simulink model "CAN_Communication"  (Simulink 8.3)
settings: Solver=ode1  StartTime=0.0  StopTime=Inf  FixedStep=0.001  RelTol=1e-3
PostLoadFcn:
  | , if any(exist('dsrtsu_mdlpostloadfcn', 'file') == [2, 3, 6]), try dsrtsu_mdlpostloadfcn('Execute', bdroot); catch fprintf('Error in PostLoadFcn (dsrtsu_mdlpostloadfcn) for model "%s":\n %s\n', bdroot, lasterr); end, end,
undefined symbols (not defined in the file or in its folder): rticanmm_blockfcn, rticanmm_initfcn
libraries: rtimmsu_dsrtlib x2
settings Model: DSRTSU_INTERNAL_RTI_VER=440  DSRTSU_INTERNAL_RTI_TYPE=rti1401  RTICANMMDATA=struct('GeneralSetupData',struct('modelroot','C:\Users\Sebastian\Desktop\DBC_Files','generalsettings',struct('filesettings',struct('destfolder',struct('Name','RTICANMM_FILES','Check',1),'buildfolder',struct('Name','.','Check',1),'AbsDestfolder',struct('Name','C:\Users\Sebastian\Desktop\DBC_Files\RTICANMM_FILES'),'AbsBuildfolder',struct('Name','C:\Users\Sebastian\Desktop\DBC_Files'))),'options',struct('addpaths',1,'rmpaths',1,'addtrcexclusion',logical(1),'cannavigator',struct('checkmonitoring',0),'show_usrtrc',0,'use_usrtrc',0,'addpath2usrmk',1),'advanced',struct('options',[1 1 1 1 1 1 1 1 1 1 1 1 1 1 1 1 1 1 1 1 1 1 1 1 1 1 1 1 1 1 1 1 1 1 1 1 1 1 1 1 1 1 1 1 1 1 1 1 1 1 1 1 1 1 1 1 1 1 1 1 1 1 1 1 1 1 1 1 1 1 1 1 1 1 1 1 1 1 1 1 1 1 1 1 1 1 1 1 1 1 1 1 1 1 1 1 1 1 1 1]),'MPSetup',{{}},'modelname','CAN_Communication','blockdata',struct('generalsettings',struct('filesettings',struct('destfolder',struct('Name','.','Check',1),'AbsDestfolder',struct('Name','T:\TOOL_SOURCES\CANnedy\m'),'buildfolder',struct('Name','.','Check',1),'AbsBuildfolder',struct('Name','C:\MATLAB6p5\work'))),'options',struct('addpaths',1,'rmpaths',1,'addpath2usrmk',1),'modelname','rticanmmlib','modelroot','T:\TOOL_SOURCES\CANnedy\m'),'MMType','RTICANMM','block',['CAN_Communication/RTICANMM' char(10) 'GeneralSetup'],'RTI',struct('Type','RTI1401','Ver','7.2','Date','02-May-2014'),'version','3.0.735671.4434490741','userdata',struct('HostServiceChannelID',{{'Controller1'}})))  DSRTSU_INTERNAL_RTIFPGA=30  Creator=Sebastian  LastModifiedBy=Sebastian  BufferReuse=off
settings DataIOCC: SignalLoggingSaveFormat=Dataset
settings OptimizationCC: BlockReduction=off  OptimizeBlockIOStorage=off  BufferReuse=off  GlobalBufferReuse=off  ExpressionFolding=off  LocalBlockOutputs=off
settings DebuggingCC: StateNameClashWarn=none
settings HardwareCC: ProdIntDivRoundTo=Zero  ProdEndianess=BigEndian  ProdHWDeviceType=Generic->Custom  TargetIntDivRoundTo=Zero  TargetEndianess=BigEndian  TargetHWDeviceType=Generic->Custom
settings RTWCC: SystemTargetFile=rti1401.tlc  MakeCommand=make_rti  TemplateMakefile=rti1401.tmf  Description=dSPACE DS1401 Hardware Platform  ProcessScript=rti1401_make_rtw_hook
settings STFCustomTargetCC: ParMdlRefBuildCompliant=on  GeneratePreprocessorConditionals=Disable all  SystemTargetFile=rti1401.tlc
settings GRTTargetCC: CompOptLevelCompliant=off  ConcurrentExecutionCompliant=off  MatFileLogging=off  CPPClassGenCompliant=off  ExtModeMexFile=noextcomm
settings CustomProperty: DataType=RTWOptions_EnumType_C__Program Files_dSPACE RCPHIL 2014-A_MATLAB_RTI_RTI1401_TLC_rti1401_1InitialSimState  Value=RUN
settings EnumStrPairs: String=RUN

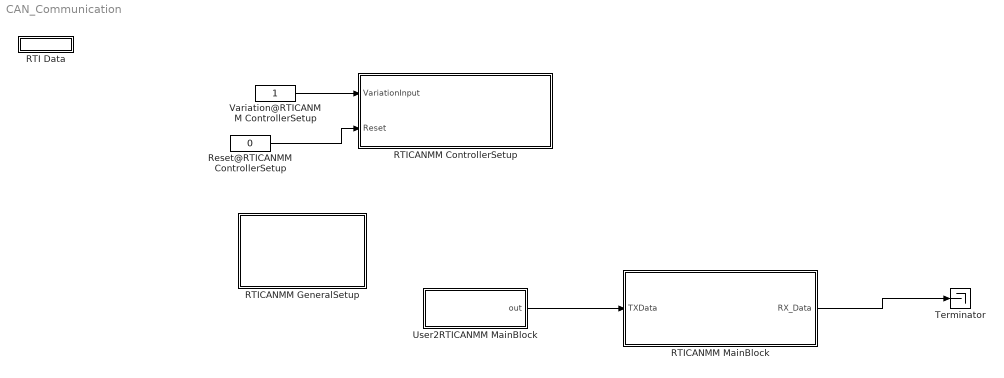
== system CAN_Communication ==
  RTI Data : Subsystem  Tag=struct('RTIDataServer',struct('RTIDataServerVs','2','RTIModelDescription','struct(''main'',''CAN_Communication'',''sub'','''',''isMp'',0)'))  LoadFcn="if exist('rtidc'), try,  rtidc('DataHostBlockClbLoad', gcbh); catch, disp(['Warning: ''LoadFcn'' for RTI Data block failed: ' lasterr]); end, end,"  mask(RTI_DATA_HOST){}
      mask help:
      | RTI Data Block.
      | This block is used by RTI to store internal model-dependent data.
      | Please keep this block on the root level of the model. Deleting this block will result in data loss.
      |
      | NEVER DELETE OR COPY THIS BLOCK!
      settings: CopyFcn="if exist('rtidc'), try,  rtidc('DataHostBlockClbCopy', gcbh); catch, disp(['Warning: ''CopyFcn'' for RTI Data block failed: ' lasterr]); end, end,"  DeleteFcn="if exist('rtidc'), try,  rtidc('DataHostBlockClbDelete', gcbh); catch, disp(['Warning: ''DeleteFcn'' for RTI Data block failed: ' lasterr]); end, end,"  ModelCloseFcn="if exist('rtidc'), try,  rtidc('DataHostBlockClbModelClose', gcbh); catch, disp(['Warning: ''ModelCloseFcn'' for RTI Data block failed: ' lasterr]); end, end,"  PreSaveFcn="if exist('rtidc'), try,  rtidc('DataHostBlockClbPreSave', gcbh); catch, disp(['Warning: ''PreSaveFcn'' for RTI Data block failed: ' lasterr]); end, end,"  PostSaveFcn="if exist('rtidc'), try,  rtidc('DataHostBlockClbPostSave', gcbh); catch, disp(['Warning: ''PostSaveFcn'' for RTI Data block failed: ' lasterr]); end, end,"  NameChangeFcn="if exist('rtidc'), try,  rtidc('DataHostBlockClbNameChange', gcbh); catch, disp(['Warning: ''NameChangeFcn'' for RTI Data block failed: ' lasterr]); end, end,"
      mask Help:
      | RTI Data Block.
      | This block is used by RTI to store internal model-dependent data.
      | Please keep this block on the root level of the model. Deleting this block will result in data loss.
      | 
      | NEVER DELETE OR COPY THIS BLOCK!
      mask Display:
      | text(0.5, 0.5, 'RTI Data', 'HorizontalAlignment', 'center');
      | plot([1 0]);
  RTICANMM ControllerSetup : Subsystem  InitFcn=rticanmm_blockfcn('InitFcn', 'CANnedySetup', gcb)  ClipboardFcn=rticanmm_blockfcn('ClipboardFcn', 'CANnedySetup', gcb)  mask(RTICANMM){DSProperties=struct('RTI',struct('Version',uint32(1),'BlockType',struct('isSLSource',uint8(1),'isSLSink',uint8(1),'isHWSource',uint8(0),'isHWSink',uint8(0),'isSetup',uint8(0),'isInline',uint8(1),'isNonInline',uint8(0),'isInterrupt',uint8(0),'isChannelwise',uint8(0)),'IOBoardType','RTICANMM','UnitType','RTICANMM','Identifier','BUSSETUP','DialogType','SL','BlockSet','RTICANMM','SlaveProcessor','CAN')), CANMMProperties=struct('cannedy',struct('data',struct('options',struct('controllername','Controller1','controllernameautomatic',[],'loglevel','0','checkrealtime',0,'checkchangebaudrate',0,'sampletime','1.000','CANControllerStatus',0,'NumberofStuffErr',0,'NumberofFormErr',0,'NumberofAckErr',0,'NumberofBit0Err',0,'NumberofsuccrecRX',0,'Numberofsuccsent',0,'NumberofBit1Err',0,'NumberofCRCErr',0,'NumberoflostRX',0,'Busoff',0,'Busload',0,'OperationPending',0,'TxRetryCount',3,'addtrcexclusion',logical(1),'cannavigator',struct('checkmonitoring',0,'checkinternmonitoring',0),'show_usrtrc',0,'use_usrtrc',0),'modelroot','C:\Users\Sebastian\Desktop\DBC_Files','generalsettings',struct('setupdata',struct('board',['CAN Type 1'],'boardno',1,'channelno',1,'Type','STD','transceiver','ISO11898-2','busconfig','0x0','feedthrough','false','resistance',struct('r120',1,'roff',0,'r16',1,'r10',0),'baudrate','500','Frequency',[24 36],'samplemode',1,'commChannelTJA1041',6,'config',struct('standard',1,'advanced',0,'register',struct('btr0','0xC0','btr1','0x6F','sp','70','sjw','3','tseg1','15','tseg2','6','brp','0','smpl','0','btr0_36','0x41','btr1_36','0x1E','sp_36','88','sjw_36','1','tseg1_36','14','tseg2_36','1','brp_36','1','smpl_36','0','btr0_64','0x43','btr1_64','0x1C','sp_64','87','sjw_64','1','tseg1_64','12','tseg2_64','1','brp_64','3','smpl_64','0')),'channelcfg',struct('INTENDISABLE','CAN_INT_DISABLE','intenable',0),'SETUPID','RTICANMM_Controller1_ID','CONTROLLER_ID','CANMM_CTL_SETUP_Controller1','mainblock_includefile','RTICANMM_SETUP_Controller1','termination','TERMINATION_ON'),'filesettings',struct('destfolder',struct('Name','RTICANMM_FILES','Check',1),'buildfolder',struct('Name','.','Check',1))),'advanced',struct('options',[1 1 1 1 1 1 1 1 1 1 1 1 1 1 1 1 1 1 1 1 1 1 1 1 1 1 1 1 1 1 1 1 1 1 1 1 1 1 1 1 1 1 1 1 1 1 1 1 1 1 1 1 1 1 1 1 1 1 1 1 1 1 1 1 1 1 1 1 1 1 1 1 1 1 1 1 1 1 1 1 1 1 1 1 1 1 1 1 1 1 1 1 1 1 1 1 1 1 1 1]),'partialnetdata',struct('switchedon',0,'format','STD','idmask',['XXXXX XXXXXXXX XXXXXXXX XXXXXXXX'],'idcode','0','idfilter','0','datamaskused',0,'datalength','0','datamask','0x0000000000000000','partialnetworkenable',0)),'blk',['CAN_Communication/RTICANMM' char(10) 'ControllerSetup'],'allgeneratedfiles',{{'C:\Users\Sebastian\Desktop\DBC_Files\RTICANMM_FILES\RTICANMM_SETUP_Controller1.c','C:\Users\Sebastian\Desktop\DBC_Files\RTICANMM_FILES\RTICANMM_SETUP_Controller1.h','c:\users\sebastian\desktop\dbc_files\rticanmm_files\rticanmm_setup_controller1.mexw64'}},'ismp',logical(0),'BlockDataVersion','0.6.0','recreate',0),'CANnedynew',0,'CANnedySettings','Controller1','GeneratedFiles',{{'C:\Users\Sebastian\Desktop\DBC_Files\RTICANMM_FILES\RTICANMM_SETUP_Controller1.c','C:\Users\Sebastian\Desktop\DBC_Files\RTICANMM_FILES\RTICANMM_SETUP_Controller1.h','c:\users\sebastian\desktop\dbc_files\rticanmm_files\rticanmm_setup_controller1.mexw64'}},'SFCN','RTICANMM_SETUP_Controller1.c','HostService',struct('Tags',struct('DATA','RTICANMM_MonitorData','Enable','CANMMMonitor_Controller1','TimeStamp','MonitoringTimeStamp_Controller1'),'DATA',struct('Length',4),'Info',struct('Desc',{'ID','Service','Data1','Data2'}),'Names',struct('Enable','Monitoring_Enable','TimeStamp','Monitoring_TimeStamp'),'ChannelID',1)), CANMMType=CANnedySetup, CANMMFolder=C:\Users\Sebastian\Desktop\DBC_Files, CANMMDestFolder=RTICANMM_FILES, CANMMSettings=Controller1, CANMMSFcn=RTICANMM_SETUP_Controller1, CANMMBoard=DS1401, CANMMBoardNum=1, CANMMChannel=1}
      settings: AttributesFormatString=%<CANMMSettings>: %<CANMMBoard>_B%<CANMMBoardNum>_C%<CANMMChannel>  CopyFcn=rticanmm_blockfcn('CopyFcn', 'CANnedySetup', gcb)  DeleteFcn=rticanmm_blockfcn('DeleteFcn', 'CANnedySetup', gcb)  ModelCloseFcn=rticanmm_blockfcn('ModelCloseFcn', 'CANnedySetup', gcb)  NameChangeFcn=rticanmm_blockfcn('NameChangeFcn', 'CANnedySetup', gcb)  OpenFcn=try, rticanmm_setup_gui('create',gcb); ; catch,errordlg({lasterr, '','Please check your RTI installation.'},['Error: ' upper(bdroot)], 'replace'); end  MoveFcn=rticanmm_blockfcn('MoveFcn', 'CANnedySetup', gcb)
      mask Help: eval('rticanmm_quickstart(''create'', gcb);', 'disp(lasterr);')
      mask Display:
      | disp('RTI CAN\nMultiMessage\nControllerSetup')
      | 
      | port_label('input', 1 , 'Variation')
      | port_label('input', 2 , 'Reset')
  RTICANMM GeneralSetup : Subsystem  InitFcn=rticanmm_initfcn(gcb, 'CANnedySettings')  ClipboardFcn=rticanmm_blockfcn('ClipboardFcn', 'CANnedySettings', gcb)  mask(RTICANMM){DSProperties=struct('RTI',struct('Version',uint32(1),'BlockType',struct('isSLSource',uint8(1),'isSLSink',uint8(1),'isHWSource',uint8(0),'isHWSink',uint8(0),'isSetup',uint8(0),'isInline',uint8(1),'isNonInline',uint8(0),'isInterrupt',uint8(0),'isChannelwise',uint8(0)),'IOBoardType','RTICANMM','UnitType','RTICANMM','Identifier','GENERALSETUP','DialogType','SL','BlockSet','RTICANMM','SlaveProcessor','CAN')), CANMMDestFolder=RTICANMM_FILES, CANMMBuildDir=., CANMMAddPaths=on, CANMMAddpathUserMake=on, CANMMRemovePathOnclose=on, CANMMType=CANnedySettings, CANMMProperties=struct('modelroot','C:\Users\Sebastian\Desktop\DBC_Files','generalsettings',struct('filesettings',struct('destfolder',struct('Name','RTICANMM_FILES','Check',1),'buildfolder',struct('Name','.','Check',1),'AbsDestfolder',struct('Name','C:\Users\Sebastian\Desktop\DBC_Files\RTICANMM_FILES'),'AbsBuildfolder',struct('Name','C:\Users\Sebastian\Desktop\DBC_Files'))),'options',struct('addpaths',1,'rmpaths',1,'addtrcexclusion',logical(1),'cannavigator',struct('checkmonitoring',0),'show_usrtrc',0,'use_usrtrc',0,'addpath2usrmk',1),'advanced',struct('options',[1 1 1 1 1 1 1 1 1 1 1 1 1 1 1 1 1 1 1 1 1 1 1 1 1 1 1 1 1 1 1 1 1 1 1 1 1 1 1 1 1 1 1 1 1 1 1 1 1 1 1 1 1 1 1 1 1 1 1 1 1 1 1 1 1 1 1 1 1 1 1 1 1 1 1 1 1 1 1 1 1 1 1 1 1 1 1 1 1 1 1 1 1 1 1 1 1 1 1 1]),'MPSetup',{{}},'modelname','CAN_Communication','blockdata',struct('generalsettings',struct('filesettings',struct('destfolder',struct('Name','.','Check',1),'AbsDestfolder',struct('Name','T:\TOOL_SOURCES\CANnedy\m'),'buildfolder',struct('Name','.','Check',1),'AbsBuildfolder',struct('Name','C:\MATLAB6p5\work'))),'options',struct('addpaths',1,'rmpaths',1,'addpath2usrmk',1),'modelname','rticanmmlib','modelroot','T:\TOOL_SOURCES\CANnedy\m'),'MMType','RTICANMM','block',['CAN_Communication/RTICANMM' char(10) 'GeneralSetup'],'RTI',struct('Type','RTI1401','Ver','7.2','Date','02-May-2014'),'version','3.0.735671.4434490741','userdata',struct('HostServiceChannelID',{{'Controller1'}}))}
      mask prompts: CANMMDestFolder "Destination Folder for generated Files:"; CANMMBuildDir "Build Directory (*_usr.mk, *_usr.trc)"; CANMMAddPaths "Add Paths automatically"; CANMMAddpathUserMake "Add Paths to UserMake-File"; CANMMRemovePathOnclose "Remove added Path on ModelClose"
      mask init:
      | rticanmm_initfcn(gcb,'CANnedyGeneralSettings')
      settings: CopyFcn=rticanmm_blockfcn('CopyFcn', 'CANnedySettings', gcb)  DeleteFcn=rticanmm_blockfcn('DeleteFcn', 'CANnedySettings', gcb)  ModelCloseFcn=rticanmm_blockfcn('CloseFcn', 'CANnedyGeneralSettings', gcb)  NameChangeFcn=rticanmm_blockfcn('NameChangeFcn', 'CANnedySettings', gcb)  OpenFcn=try, rticanmm_gs_gui('create',gcb), ; catch,errordlg({lasterr, '','Please check your RTI installation.'},['Error: ' upper(bdroot)], 'replace'); end  MoveFcn=rticanmm_blockfcn('MoveFcn', 'CANnedySettings', gcb)
      mask Help: eval('rticanmm_quickstart(''create'', gcb);', 'disp(lasterr);')
      mask Display: disp(sprintf(['RTI CAN\nMultiMessage\nGeneralSetup']))
  RTICANMM MainBlock : Subsystem  InitFcn=rticanmm_blockfcn('InitFcn', 'CANnedy', gcb)  ClipboardFcn=rticanmm_blockfcn('ClipboardFcn', 'CANnedy', gcb)  mask(RTICANMM){DSProperties=struct('RTI',struct('Version',uint32(1),'BlockType',struct('isSLSource',uint8(1),'isSLSink',uint8(1),'isHWSource',uint8(0),'isHWSink',uint8(0),'isSetup',uint8(0),'isInline',uint8(1),'isNonInline',uint8(0),'isInterrupt',uint8(0),'isChannelwise',uint8(0)),'IOBoardType','RTICANMM','UnitType','RTICANMM','Identifier','Mainblock','DialogType','SL','BlockSet','RTICANMM','SlaveProcessor','CAN')), CANMMProperties=struct('RTICANMMVersion','3.0','RTICANMMVersionIntern','3.0.735671.4434490741','RTICANMMDate','02-May-2014','Settings','RTICANMM_MAIN_CAN','UserTracePath','','ModelPath','C:\Users\Sebastian\Desktop\DBC_Files','filesettings',struct('FileName','AngleSpeed.dbc','IsRelative',1,'ClusterId',1,'ClusterList',{{'default'}},'destfolder',struct('Name','RTICANMM_FILES','Check',1),'buildfolder',struct('Name','.','Check',1),'onlyfreerawcapture',0,'overlapping2variant',0),'onlyfreerawcapture',0,'Board',['CAN Type 1'],'BoardNum','1','ChannelNum','1','Variation','1','SetupId','Controller1','MARK',['719753203727948A60AC430329C9D5';'48A0AF194FAB6FB27E8338C8940826';'1300DB01B7EF55C98D2EBFEB02253B';'5389981ECFCAA947711D2E68ACED04';'4C61CF917CD092FC8858619250CB50'],'date','13-Jan-2015','clock',['13.01.2015 19:24:34'],'recreate',0,'RTIVER','RTI1401','j1939',0,'TRC',struct('include',1),'rtsupport',struct('XMLFile','C:\Users\Sebastian\Desktop\DBC_Files\RTICANMM_FILES\RTICANMM_MAIN_CAN.xml','DBCXML',struct('Path','C:\Users\Sebastian\Desktop\DBC_Files\RTICANMM_FILES\RTICANMM_MAIN_CAN_dbc.xml','support',1,'Name','AngleSpeed.dbc','Date',['11-Dez-2014 10:18:45'],'Type','extended','DBCSupport','ON'))), CANMMType=CANnedy, CANMMUserTraceMerged=off, CANMMUserTracePath=, CANMMChannelNum=1, CANMMBoardNum=1, CANMMDestFolder=RTICANMM_FILES, CANMMFolder=., CANMMSetupId=Controller1, CANMMsave2mat=['719753203727948A60AC430329C9D5';'48A0AF194FAB6FB27E8338C8940826';'1300DB01B7EF55C98D2EBFEB02253B';'5389981ECFCAA947711D2E68ACED04';'4C61CF917CD092FC8858619250CB50'], CANMMName=CAN, CANMMSettings=RTICANMM_MAIN_CAN, CANMMIntermediateTag=RTICANMM_MAIN_CAN_intermediate, CANMMsfcnname=RTICANMM_MAIN_CAN}
      mask init:
      | rticanmm_initfcn(gcb, CANMMType, CANMMsfcnname)
      settings: AttributesFormatString=Controller1[CAN]: DS1401_B1_C1_V1  CopyFcn=rticanmm_blockfcn('CopyFcn', 'CANnedy', gcb)  DeleteFcn=rticanmm_blockfcn('DeleteFcn', 'CANnedy', gcb)  ModelCloseFcn=rticanmm_blockfcn('ModelCloseFcn', 'CANnedy', gcb)  NameChangeFcn=rticanmm_blockfcn('NameChangeFcn', 'CANnedy', gcb)  OpenFcn=try, rticanmm_main_gui('create',gcb); ; catch,errordlg({lasterr, '','Please check your RTI installation.'},['Error: ' upper(bdroot)], 'replace'); end  MoveFcn=rticanmm_blockfcn('MoveFcn', 'CANnedy', gcb)
      mask Help: eval('rticanmm_quickstart(''create'', gcb);', 'disp(lasterr);')
      mask Display:
      | disp(sprintf('RTI CAN\nMultiMessage\nMainSetup'))
      | port_label('input', 1, 'TX Data')
      | port_label('output', 1, 'RX Data')
  Reset@RTICANMM ControllerSetup : Constant  Value=0  OutDataTypeStr=boolean
  Terminator : Terminator
  User2RTICANMM MainBlock : Subsystem
      mask Display: disp('Mapping\nto RTICANMM')
  Variation@RTICANMM ControllerSetup : Constant  OutDataTypeStr=uint8
  wires:
  Variation@RTICANMM ControllerSetup/1 -> RTICANMM ControllerSetup/1(VariationInput)
  Reset@RTICANMM ControllerSetup/1 -> RTICANMM ControllerSetup/2(Reset)
  User2RTICANMM MainBlock/1(out) -> RTICANMM MainBlock/1(TXData)
  RTICANMM MainBlock/1(RX_Data) -> Terminator/1

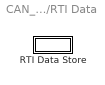
== system CAN_Communication/RTI Data ==
  RTI Data Store : Subsystem  Tag="struct('private',struct('version',struct('dsVer',uint32(2),'dsVerCreation',uint32(2),'RTI',struct('ver','7.2','type','RTI1401')),'access',struct('type','Model','isPerm',1,'created',['13-Jan-2015 19:18:04'],'modified',['13-Jan-2015 20:17:45'],'location','')),'public',struct('main',struct('data',[]),'sub',struct('name',{{'CAN_Communication'}},'data',{{struct('TH',struct('thTaskInfo',struct('taskType',{'TIMER','HWINT','TMRINT','SWINT','GLINT'},'tasksNumOf',{1,0,0,0,0},'srcIds',{{'TIMERA'},{},{},{},{}},'taskNames',{{['Timer Task 1']},{},{},{},{}})),'th_tc',struct('dataType','TASK','taskGroupId','','taskGroupList',{{}},'taskSchedulingPolicy','FCFS','taskType','TIMER','blkh',-1,'srcId','TIMERA','srcSgnName',['Timer A interrupt'],'srcCpuName','','taskName',['Timer Task 1  [0.001] s'],'taskNameDisplayExt','','smplTime',0.001,'smplTimeOffs',0,'hasFixedPriority',0,'priority',1,'hasFixedOvc',0,'ovcType',1,'ovcMax',1),'tc_th',struct('dataType','TASK','taskGroupId','','taskGroupList',{{}},'taskSchedulingPolicy','FCFS','taskType','TIMER','blkh',-1,'srcId','TIMERA','srcSgnName',['Timer A interrupt'],'srcCpuName','','taskName',['Timer Task 1  [0.001] s'],'taskNameDisplayExt','','smplTime',0.001,'smplTimeOffs',0,'hasFixedPriority',0,'priority',1,'hasFixedOvc',0,'ovcType',1,'ovcMax',1))}})))"  mask(RTI_DATA_STORE){}
      mask help:
      | RTI Data Store Block. This block is used by RTI to store internal model dependent data. Deleting this block will result in data loss.
      |
      | NEVER DELETE, COPY, OR MODIFY THIS BLOCK!
      mask Help:
      | RTI Data Store Block. This block is used by RTI to store internal model dependent data. Deleting this block will result in data loss.
      | 
      | NEVER DELETE, COPY, OR MODIFY THIS BLOCK!
      mask Display: text(0.5, 0.5, ' ', 'HorizontalAlignment', 'center');

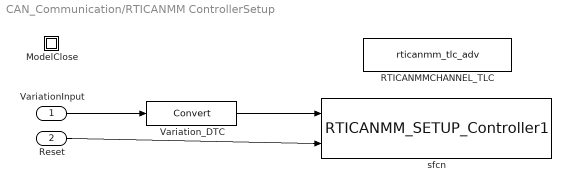
== system CAN_Communication/RTICANMM ControllerSetup ==
  VariationInput : Inport
  Reset : Inport  Port=2
  ModelClose : Subsystem  mask(RTICANMMModelClose){}
  RTICANMMCHANNEL_TLC : S-Function  FunctionName=rticanmm_tlc_adv  Parameters=1401,1,1,0,500,'unused'  EnableBusSupport=off  mask(RTICANMMCHANNEL_TLC){}
  Variation_DTC : DataTypeConversion  SaturateOnIntegerOverflow=on  RndMeth=Zero
  sfcn : S-Function  InitFcn=rticanmm_initfcn(gcb, 'SFCNs')  FunctionName=RTICANMM_SETUP_Controller1  EnableBusSupport=off
      mask init:
      | rticanmm_initfcn(gcb, 'SFCNs')
  wires:
  Reset/1 -> sfcn/2
  VariationInput/1 -> Variation_DTC/1
  Variation_DTC/1 -> sfcn/1

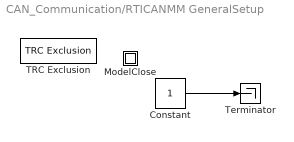
== system CAN_Communication/RTICANMM GeneralSetup ==
  Constant : Constant
  ModelClose : Subsystem  mask(RTICANMMModelClose){}
  TRC Exclusion : rtimmsu_dsrtlib/TRC Exclusion
  Terminator : Terminator
  wires:
  Constant/1 -> Terminator/1

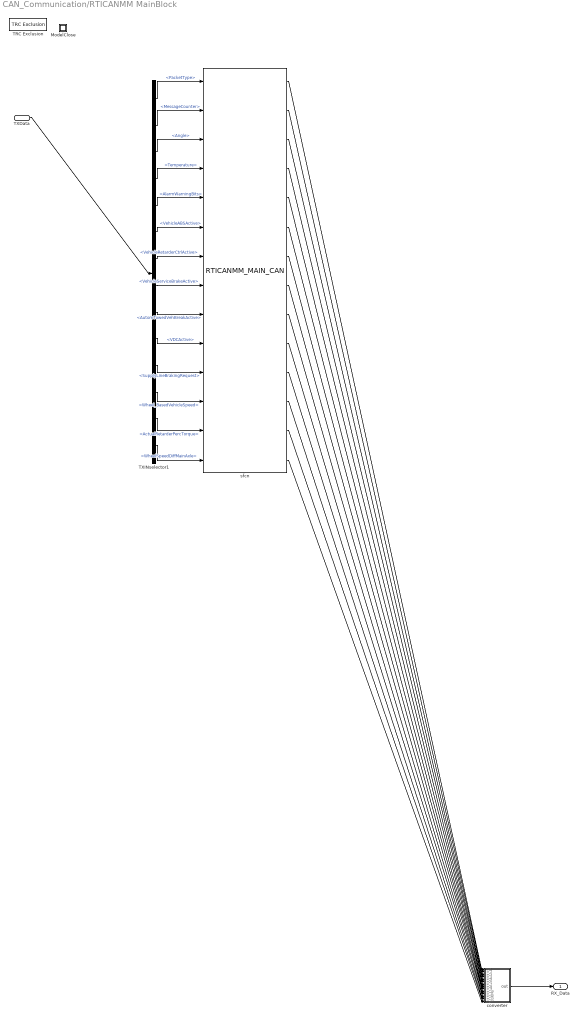
== system CAN_Communication/RTICANMM MainBlock ==
  TXData : Inport
  ModelClose : Subsystem  mask(RTICANMMModelClose){}
  TRC Exclusion : rtimmsu_dsrtlib/TRC Exclusion
  TXINselector1 : BusSelector  OutputSignals=AngleSensor.PacketType,AngleSensor.MessageCounter,AngleSensor.Angle,AngleSensor.Temperature,AngleSensor.AlarmWarningBits,ISO11992_EBS21.VehicleABSActive,ISO11992_EBS21.VehicleRetarderCtrlActive,ISO11992_EBS21.VehicleServiceBrakeActive,ISO11992_EBS21.AutomTowedVehBreakActive,ISO11992_EBS21.VDCActive,ISO11992_EBS21.SupplyLineBrakingRequest,ISO11992_EBS21.Wheel_BasedVehicleSpeed,ISO11992_EBS21.ActualRetarderPercTorque,ISO11992_EBS21.WheelSpeedDiffMainAxle
  converter : Subsystem  mask(CANnedyVector2Bus){}
      mask help: Do not change.
      mask Display: disp('Vector to\nBus')
  sfcn : S-Function  InitFcn=rticanmm_initfcn(gcb, 'SFCNs')  FunctionName=RTICANMM_MAIN_CAN  EnableBusSupport=off
      mask init:
      | rticanmm_initfcn(gcb, 'SFCNs')
  RX_Data : Outport
  wires:
  TXData/1 -> TXINselector1/1
  TXINselector1/1 -> sfcn/1  "<PacketType>"
  TXINselector1/2 -> sfcn/2  "<MessageCounter>"
  TXINselector1/3 -> sfcn/3  "<Angle>"
  TXINselector1/4 -> sfcn/4  "<Temperature>"
  TXINselector1/5 -> sfcn/5  "<AlarmWarningBits>"
  TXINselector1/6 -> sfcn/6  "<VehicleABSActive>"
  TXINselector1/7 -> sfcn/7  "<VehicleRetarderCtrlActive>"
  TXINselector1/8 -> sfcn/8  "<VehicleServiceBrakeActive>"
  TXINselector1/9 -> sfcn/9  "<AutomTowedVehBreakActive>"
  TXINselector1/10 -> sfcn/10  "<VDCActive>"
  TXINselector1/11 -> sfcn/11  "<SupplyLineBrakingRequest>"
  TXINselector1/12 -> sfcn/12  "<Wheel_BasedVehicleSpeed>"
  TXINselector1/13 -> sfcn/13  "<ActualRetarderPercTorque>"
  TXINselector1/14 -> sfcn/14  "<WheelSpeedDiffMainAxle>"
  converter/1(out) -> RX_Data/1
  sfcn/1 -> converter/1(in_1)
  sfcn/2 -> converter/2(in_2)
  sfcn/3 -> converter/3(in_3)
  sfcn/4 -> converter/4(in_4)
  sfcn/5 -> converter/5(in_5)
  sfcn/6 -> converter/6(in_6)
  sfcn/7 -> converter/7(in_7)
  sfcn/8 -> converter/8(in_8)
  sfcn/9 -> converter/9(in_9)
  sfcn/10 -> converter/10(in_10)
  sfcn/11 -> converter/11(in_11)
  sfcn/12 -> converter/12(in_12)
  sfcn/13 -> converter/13(in_13)
  sfcn/14 -> converter/14(in_14)

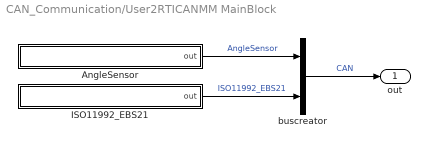
== system CAN_Communication/User2RTICANMM MainBlock ==
  AngleSensor : Subsystem
  ISO11992_EBS21 : Subsystem
  buscreator : BusCreator  Inputs=2
  out : Outport
  wires:
  AngleSensor/1(out) -> buscreator/1  "AngleSensor"
  ISO11992_EBS21/1(out) -> buscreator/2  "ISO11992_EBS21"
  buscreator/1 -> out/1  "CAN"

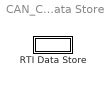
== system CAN_Communication/RTI Data/RTI Data Store ==
  RTI Data Store : Subsystem  mask(RTI_DATA_STORE){}
      mask help:
      | RTI Data Store Block. This block is used by RTI to store internal model dependent data. Deleting this block will result in data loss.
      |
      | NEVER DELETE, COPY, OR MODIFY THIS BLOCK!
      mask Help:
      | RTI Data Store Block. This block is used by RTI to store internal model dependent data. Deleting this block will result in data loss.
      | 
      | NEVER DELETE, COPY, OR MODIFY THIS BLOCK!
      mask Display: text(0.5, 0.5, ' ', 'HorizontalAlignment', 'center');

== system CAN_Communication/RTICANMM ControllerSetup/ModelClose ==

== system CAN_Communication/RTICANMM GeneralSetup/ModelClose ==

== system CAN_Communication/RTICANMM MainBlock/ModelClose ==

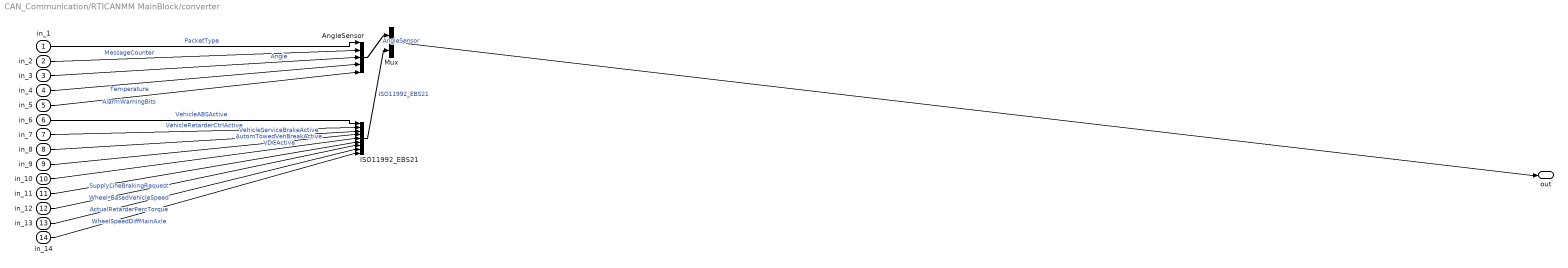
== system CAN_Communication/RTICANMM MainBlock/converter ==
  in_1 : Inport
  in_2 : Inport  Port=2
  in_3 : Inport  Port=3
  in_4 : Inport  Port=4
  in_5 : Inport  Port=5
  in_6 : Inport  Port=6
  in_7 : Inport  Port=7
  in_8 : Inport  Port=8
  in_9 : Inport  Port=9
  in_10 : Inport  Port=10
  in_11 : Inport  Port=11
  in_12 : Inport  Port=12
  in_13 : Inport  Port=13
  in_14 : Inport  Port=14
  AngleSensor : BusCreator  Inputs=5
  ISO11992_EBS21 : BusCreator  Inputs=9
  Mux : BusCreator  Inputs=2
  out : Outport
  wires:
  in_1/1 -> AngleSensor/1  "PacketType"
  AngleSensor/1 -> Mux/1  "AngleSensor"
  in_2/1 -> AngleSensor/2  "MessageCounter"
  in_3/1 -> AngleSensor/3  "Angle"
  in_4/1 -> AngleSensor/4  "Temperature"
  in_5/1 -> AngleSensor/5  "AlarmWarningBits"
  in_6/1 -> ISO11992_EBS21/1  "VehicleABSActive"
  ISO11992_EBS21/1 -> Mux/2  "ISO11992_EBS21"
  in_7/1 -> ISO11992_EBS21/2  "VehicleRetarderCtrlActive"
  in_8/1 -> ISO11992_EBS21/3  "VehicleServiceBrakeActive"
  in_9/1 -> ISO11992_EBS21/4  "AutomTowedVehBreakActive"
  in_10/1 -> ISO11992_EBS21/5  "VDCActive"
  in_11/1 -> ISO11992_EBS21/6  "SupplyLineBrakingRequest"
  in_12/1 -> ISO11992_EBS21/7  "Wheel_BasedVehicleSpeed"
  in_13/1 -> ISO11992_EBS21/8  "ActualRetarderPercTorque"
  in_14/1 -> ISO11992_EBS21/9  "WheelSpeedDiffMainAxle"
  Mux/1 -> out/1

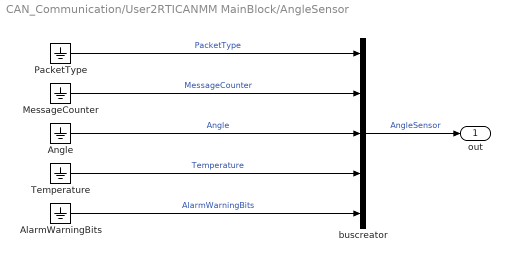
== system CAN_Communication/User2RTICANMM MainBlock/AngleSensor ==
  AlarmWarningBits : Ground
  Angle : Ground
  MessageCounter : Ground
  PacketType : Ground
  Temperature : Ground
  buscreator : BusCreator  Inputs=5
  out : Outport
  wires:
  buscreator/1 -> out/1  "AngleSensor"
  PacketType/1 -> buscreator/1  "PacketType"
  MessageCounter/1 -> buscreator/2  "MessageCounter"
  Angle/1 -> buscreator/3  "Angle"
  Temperature/1 -> buscreator/4  "Temperature"
  AlarmWarningBits/1 -> buscreator/5  "AlarmWarningBits"

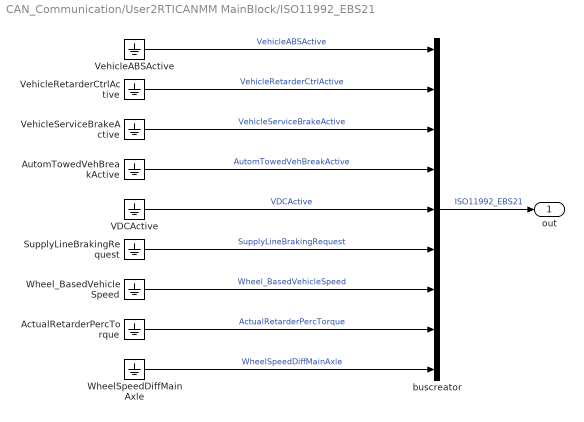
== system CAN_Communication/User2RTICANMM MainBlock/ISO11992_EBS21 ==
  ActualRetarderPercTorque : Ground
  AutomTowedVehBreakActive : Ground
  SupplyLineBrakingRequest : Ground
  VDCActive : Ground
  VehicleABSActive : Ground
  VehicleRetarderCtrlActive : Ground
  VehicleServiceBrakeActive : Ground
  WheelSpeedDiffMainAxle : Ground
  Wheel_BasedVehicleSpeed : Ground
  buscreator : BusCreator  Inputs=9
  out : Outport
  wires:
  buscreator/1 -> out/1  "ISO11992_EBS21"
  VehicleABSActive/1 -> buscreator/1  "VehicleABSActive"
  VehicleRetarderCtrlActive/1 -> buscreator/2  "VehicleRetarderCtrlActive"
  VehicleServiceBrakeActive/1 -> buscreator/3  "VehicleServiceBrakeActive"
  AutomTowedVehBreakActive/1 -> buscreator/4  "AutomTowedVehBreakActive"
  VDCActive/1 -> buscreator/5  "VDCActive"
  SupplyLineBrakingRequest/1 -> buscreator/6  "SupplyLineBrakingRequest"
  Wheel_BasedVehicleSpeed/1 -> buscreator/7  "Wheel_BasedVehicleSpeed"
  ActualRetarderPercTorque/1 -> buscreator/8  "ActualRetarderPercTorque"
  WheelSpeedDiffMainAxle/1 -> buscreator/9  "WheelSpeedDiffMainAxle"

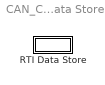
== system CAN_Communication/RTI Data/RTI Data Store/RTI Data Store ==
  RTI Data Store : Subsystem  mask(RTI_DATA_STORE){}
      mask help:
      | RTI Data Store Block. This block is used by RTI to store internal model dependent data. Deleting this block will result in data loss.
      |
      | NEVER DELETE, COPY, OR MODIFY THIS BLOCK!
      mask Help:
      | RTI Data Store Block. This block is used by RTI to store internal model dependent data. Deleting this block will result in data loss.
      | 
      | NEVER DELETE, COPY, OR MODIFY THIS BLOCK!
      mask Display: text(0.5, 0.5, ' ', 'HorizontalAlignment', 'center');

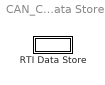
== system CAN_Communication/RTI Data/RTI Data Store/RTI Data Store/RTI Data Store ==
  RTI Data Store : Subsystem  mask(RTI_DATA_STORE){}
      mask help:
      | RTI Data Store Block. This block is used by RTI to store internal model dependent data. Deleting this block will result in data loss.
      |
      | NEVER DELETE, COPY, OR MODIFY THIS BLOCK!
      mask Help:
      | RTI Data Store Block. This block is used by RTI to store internal model dependent data. Deleting this block will result in data loss.
      | 
      | NEVER DELETE, COPY, OR MODIFY THIS BLOCK!
      mask Display: text(0.5, 0.5, ' ', 'HorizontalAlignment', 'center');

== system CAN_Communication/RTI Data/RTI Data Store/RTI Data Store/RTI Data Store/RTI Data Store ==
